simulink model "ext_steer_all"  (Simulink 8.8)
settings: Solver=ode45  StartTime=0  StopTime=110  FixedStep=0.002  RelTol=1e-3  AbsTol=1e-6
libraries: Solver_SF x1
settings Model: Creator=ywata  LastModifiedBy=mkhan  ExtModeTrigMode=oneshot  ExtModeArmWhenConnect=off
settings DataIOCC: LimitDataPoints=off  SignalLoggingName=sigsOut
settings OptimizationCC: BlockReduction=off  BooleanDataType=off
settings DebuggingCC: SaveWithParameterizedLinksMsg=none  SignalResolutionControl=TryResolveAllWithWarning  MultiTaskDSMMsg=warning  MultiTaskCondExecSysMsg=none  SFExecutionAtInitializationDiag=warning
settings HardwareCC: TargetUnknown=on
settings RTWCC: TemplateMakefile=grt_vc.tmf
settings GRTTargetCC: TargetFcnLib=ansi_tfl_tmw.mat
settings ConfigComp: CovSFcnEnable=off

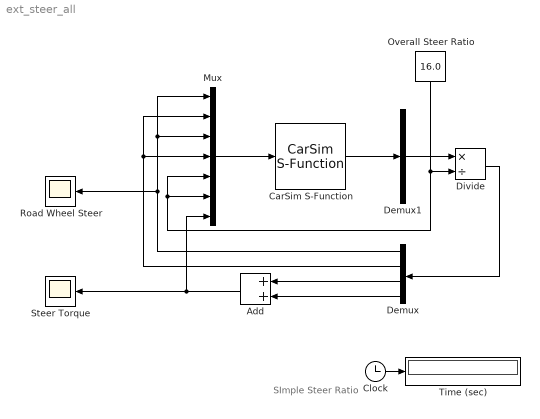
== system ext_steer_all ==
  note: SImple Steer Ratio
  Add : Sum
  CarSim S-Function : Solver_SF/CarSim S-Function  Priority=1  SIMFILE=simfile.sim  Run_RTs=off  vs_state_ind=Run  StopMode_ind=Vehicle Model
  Clock : Clock
  Demux : Demux
  Demux1 : Demux  Outputs=[4]
      settings: DisplayOption=none
  Divide : Product  Inputs=*/
  Mux : Mux  Inputs=7
  Overall Steer Ratio : Constant  Value=16.0
  Road Wheel Steer : Scope
  Steer Torque : Scope
  Time (sec) : Display
      settings: Format=bank  Decimation=100
  wires:
  Clock/1 -> Time (sec)/1
  Demux1/1 -> Divide/1
  Divide/1 -> Demux/1
  Demux/1 -> Mux/3, Mux/1, Road Wheel Steer/1
  Demux/2 -> Mux/4, Mux/2
  Overall Steer Ratio/1 -> Divide/2, Mux/6, Mux/5
  Demux/3 -> Add/1
  Demux/4 -> Add/2
  Add/1 -> Steer Torque/1, Mux/7
  CarSim S-Function/1 -> Demux1/1
  Mux/1 -> CarSim S-Function/1
